simulink model "Environment_per_immagini_TESI"  (R2023a)
settings: Solver=FixedStepAuto  StartTime=0.0  StopTime=inf  RelTol=1e-3
values from neighbouring files (symbols this model uses):
  traiettoria = [x', y']    [generatoreTraiettoria.m]    (also in generatoreTraiettoria2.m; tra3.m)
undefined symbols (not defined in the file or in its folder): a, e1_0, p, Vdes
libraries: simulink x2, rllib x1
settings Model: Creator=Luzi  LastModifiedBy=Luzi

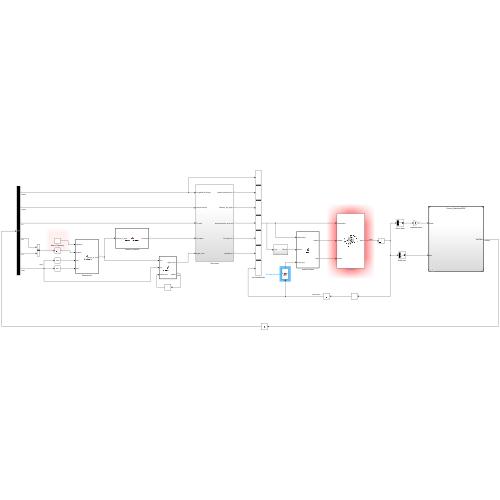
[thumbnail: Simulink's stored preview of the top-level diagram]
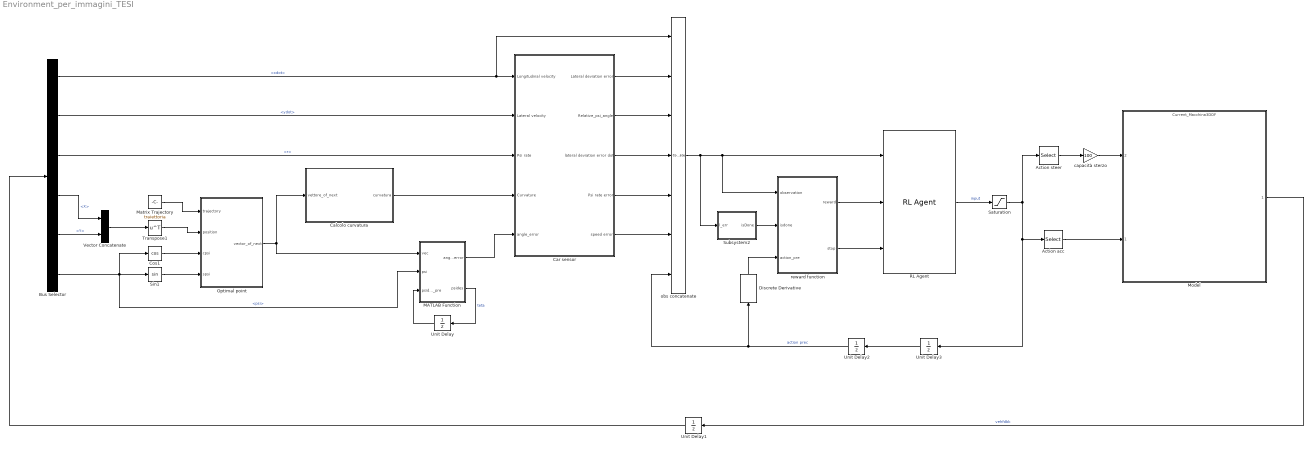
== system Environment_per_immagini_TESI ==
  Action acc : Selector  InputPortWidth=2  IndexOptions=Index vector (dialog)  Indices=2  OutputSizes=1
  Action steer : Selector  InputPortWidth=2  IndexOptions=Index vector (dialog)  Indices=1  OutputSizes=1
  Bus Selector : BusSelector  OutputSignals=BdyFrm.Cg.Vel.xdot,BdyFrm.Cg.Vel.ydot,BdyFrm.Cg.AngVel.r,InertFrm.Cg.Disp.X,InertFrm.Cg.Disp.Y,InertFrm.Cg.Ang.psi
  Calcolo curvatura : MATLAB Function  TreatAsAtomicUnit=on
  Car sensor : Subsystem
  Cos1 : Trigonometry  Operator=cos
  Discrete Derivative : simulink/Discrete/Discrete Derivative  gainval=0.1  ICPrevScaledInput=0.0  OutMin=[]  OutMax=[]  OutDataType=fixdt(1, 16)  OutScaling=2^-10  DoSatur=off
  MATLAB Function : MATLAB Function  TreatAsAtomicUnit=on
  Matrix Trajectory : Constant  Value=traiettoria  SampleTime=60
  Model : ModelReference  ModelNameDialog=Current_Macchina3DOF.slx  SimulationMode=Normal  ModelReferenceVersion=1.71
      settings: PortSchema="{\"entries\":[{\"content\":{\"sides\":[{\"content\":{\"connectorIds\":[\"In2\",\"In1\"]},\"type\":\"ConnectorPlacement.EquallySpacedRectSide\",\"uuid\":\"b5a44853-6584-4a50-847d-9a0b1c5ea9ac\"},{\"content\":{\"connectorIds\":[\"Out1\"],\"side\":\"RIGHT\"},\"type\":\"ConnectorPlacement.EquallySpacedRectSide\",\"uuid\":\"bfcb6c88-1d93-4f70-bf16-2c719fa247ba\"},{\"content\":{\"side\":\"TOP\"},\"type\":\"ConnectorPlacement.EquallySpacedRectSide\",\"uuid\":\"3385b00b-6ed4-40a5-8204-01acdd431cf5\"}]},\"type\":\"ConnectorPlacement.EquallySpacedConnector\",\"uuid\":\"3bb36942-6fbc-4d27-a33b-ca1de48b267b\"}],\"packageUris\":[\"http://schema.mathworks.com/mf0/Connector/R2020b\"],\"version\":\"1.0\"}"
  Optimal point : MATLAB Function  TreatAsAtomicUnit=on
  RL Agent : rllib/RL Agent  Agent=agent  ExternalActionAsInput=off  ProvideLastAction=off  ProvideCumRwd=off  TreatAsDirectFeedthrough=on  UseStrictObservationDataTypes=off
  Saturation : Saturate  UpperLimit=1  LowerLimit=-1
  Sin1 : Trigonometry
  Subsystem2 : Subsystem
  Transpose1 : Math  Operator=transpose
  Unit Delay{,1..3} (4 alike) : UnitDelay  SampleTime=-1  HasFrameUpgradeWarning=on
  Vector Concatenate : Concatenate
  capacità sterzo : Gain  Gain=100
  obs concatenate : Concatenate  NumInputs=7
  reward function : MATLAB Function  TreatAsAtomicUnit=on
  wires:
  Saturation/1 -> Action steer/1, Unit Delay3/1, Action acc/1
  Bus Selector/1 -> obs concatenate/1, Car sensor/1(Longitudinal velocity)  "<xdot>"
  Action steer/1 -> capacità sterzo/1
  obs concatenate/1 -> Subsystem2/1(l_err), reward function/1(observation), RL Agent/1
  RL Agent/1 -> Saturation/1  "input"
  Action acc/1 -> Model/1
  Bus Selector/2 -> Car sensor/2(Lateral velocity)  "<ydot>"
  Bus Selector/3 -> Car sensor/3(Psi rate)  "<r>"
  Calcolo curvatura/1(curvatura) -> Car sensor/4(Curvature)
  MATLAB Function/1(angle_error) -> Car sensor/5(angle_error)
  Unit Delay2/1 -> Discrete Derivative/1, obs concatenate/7  "action prec"
  Car sensor/5(speed error) -> obs concatenate/6
  Car sensor/4(Psi rate error) -> obs concatenate/5
  Car sensor/3(lateral deviation error dot) -> obs concatenate/4
  Car sensor/2(Relative_psi_angle) -> obs concatenate/3
  Car sensor/1(Lateral deviation error) -> obs concatenate/2
  MATLAB Function/2(psides) -> Unit Delay/1  "teta"
  Unit Delay/1 -> MATLAB Function/3(psides_pre)
  Optimal point/1(vector_of_next) -> Calcolo curvatura/1(vettore_of_next), MATLAB Function/1(vec)
  capacità sterzo/1 -> Model/2
  Model/1 -> Unit Delay1/1  "vehfdbk"
  Cos1/1 -> Optimal point/3(cpsi)
  Vector Concatenate/1 -> Transpose1/1
  Matrix Trajectory/1 -> Optimal point/1(trajectory)
  Bus Selector/6 -> MATLAB Function/2(psi), Sin1/1, Cos1/1  "<psi>"
  Sin1/1 -> Optimal point/4(spsi)
  Transpose1/1 -> Optimal point/2(position)
  Bus Selector/4 -> Vector Concatenate/1  "<X>"
  Bus Selector/5 -> Vector Concatenate/2  "<Y>"
  Subsystem2/1(isDone) -> reward function/2(isdone)
  reward function/2(stop) -> RL Agent/3
  reward function/1(reward) -> RL Agent/2
  Discrete Derivative/1 -> reward function/3(action_pre)
  Unit Delay1/1 -> Bus Selector/1
  Unit Delay3/1 -> Unit Delay2/1

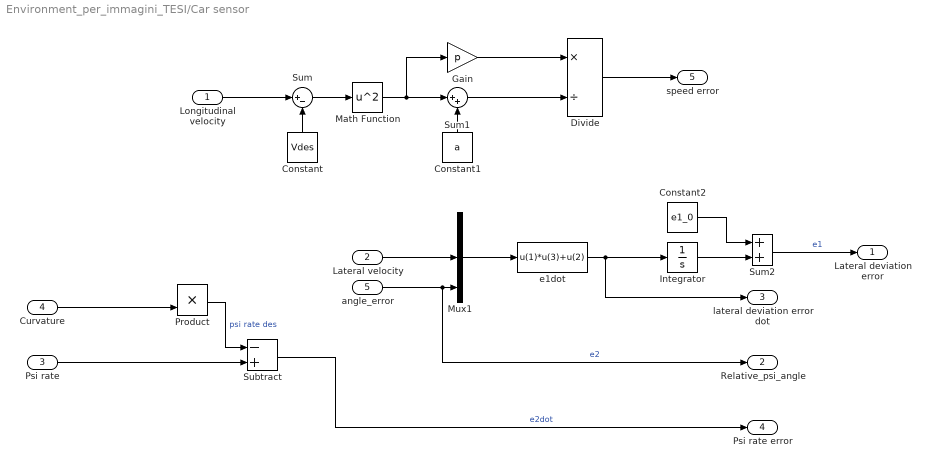
== system Environment_per_immagini_TESI/Car sensor ==
  Longitudinal velocity : Inport
  Lateral velocity : Inport  Port=2
  Psi rate : Inport  Port=3
  Curvature : Inport  Port=4
  angle_error : Inport  Port=5
  Constant : Constant  Value=Vdes
  Constant1 : Constant  Value=a
  Constant2 : Constant  Value=e1_0
  Divide : Product  Inputs=*/
  Gain : Gain  Gain=p
  Integrator : Integrator
  Math Function : Math  Operator=square
  Mux1 : Mux  Inputs=[1 1 1]
  Product : Product
  Subtract : Sum  Inputs=-+
  Sum : Sum  Inputs=|+-
  Sum1 : Sum  Inputs=|++
  Sum2 : Sum
  e1dot : Fcn  Expr=u(1)*u(3)+u(2)
  Lateral deviation error : Outport  VectorParamsAs1DForOutWhenUnconnected=off
  Relative_psi_angle : Outport  Port=2
  lateral deviation error dot : Outport  Port=3  VectorParamsAs1DForOutWhenUnconnected=off
  Psi rate error : Outport  Port=4  VectorParamsAs1DForOutWhenUnconnected=off
  speed error : Outport  Port=5
  wires:
  Curvature/1 -> Product/2
  Mux1/1 -> e1dot/1
  e1dot/1 -> lateral deviation error dot/1, Integrator/1
  Lateral velocity/1 -> Mux1/2
  Product/1 -> Subtract/1  "psi rate des"
  Psi rate/1 -> Subtract/2
  Subtract/1 -> Psi rate error/1  "e2dot"
  angle_error/1 -> Relative_psi_angle/1, Mux1/3  "e2"
  Constant/1 -> Sum/2
  Sum/1 -> Math Function/1
  Longitudinal velocity/1 -> Sum/1
  Math Function/1 -> Gain/1, Sum1/1
  Constant1/1 -> Sum1/2
  Sum1/1 -> Divide/2
  Gain/1 -> Divide/1
  Divide/1 -> speed error/1
  Integrator/1 -> Sum2/2
  Sum2/1 -> Lateral deviation error/1  "e1"
  Constant2/1 -> Sum2/1

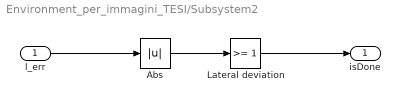
== system Environment_per_immagini_TESI/Subsystem2 ==
  l_err : Inport
  Abs : Abs  SaturateOnIntegerOverflow=off
  Lateral deviation : simulink/Logic and Bit Operations/Compare To Constant  relop=>=  const=1  OutDataTypeStr=boolean
  isDone : Outport  VectorParamsAs1DForOutWhenUnconnected=off
  wires:
  Abs/1 -> Lateral deviation/1
  l_err/1 -> Abs/1
  Lateral deviation/1 -> isDone/1

== matlab function Environment_per_immagini_TESI/MATLAB Function ==
  data: vec input; psi input; angle_error output; psides output; psides_pre input
function [angle_error,psides] = calc_angle_error(vec,psi, psides_pre)
    x1=vec(1,1);
    y1=vec(1,2);
    x3=vec(3,1);
    y3=vec(3,2);
    psides=atan2((y3-y1),(x3-x1));


     if(abs(tetapre-psides)>pi/4 && abs(tetapre-psides)<1.1*pi)%ATTENZIONE: PROVVISORIO PER RISOLVERE IL PROBLEMA DELL'INCROCIO DI TRAIETTORIE
         psides=tetapre;
     end



    angle_error=psi-psides;
    if angle_error>pi
        angle_error=angle_error-2*pi;
    elseif angle_error<-pi
        angle_error=angle_error+2*pi;
    end
end

== matlab function Environment_per_immagini_TESI/reward function ==
  data: observation input; isdone input; action_pre input; reward output; stop output
function [reward, stop] = reward(observation, isdone, action_pre)
    % Input:
    %   observation: vector containing relevant state information
    %   isdone: flag indicating whether the episode is finished
    %   action: vector representing the action taken
    %   action_d: vector representing the action derivatives
    % Output:
    %   speed_error: computed speed error based on the current velocity
    %   reward: calculated reward value considering various factors
    %   stop: flag indicating whether the episode should stop

    % Apply bonus based on lateral deviation
    
    if (e1^2 < 0.04)
        bonus_pos = 2;
    end

    if (e1^2 < 0.01)
        bonus_pos = bonus_pos + 0.5;
    end

    % Calculate the reward value
    reward = -(2 * e1^2 + 0.5*e2^2) - 50 * isdone + bonus_pos - speed_error - 0.25 * a_dot^2 - 1 * s_dot^2;

    stop = isdone;
end

%funzione countorf(x,y,z) per mappatura ricompenra e colorbar da inserire
%(nel editor matlab) per il controllo funzionalità

== matlab function Environment_per_immagini_TESI/Optimal point ==
  data: trajectory input; position input; cpsi input; spsi input; vector_of_next output
function vector_of_next  = optimalpoint(trajectory, position, cpsi, spsi)
    % Input:
    %   trajectory: Nx2 matrix representing the trajectory points
    %   position: 1x2 row vector representing the current position (xy)
    %   cpsi, spsi: components of the velocity direction
    % Output:
    %   point: 1x2 row vector representing the optimal point on the trajectory
    %   vector_of_next: 3x2 matrix containing the optimal point and the next two points

    % Initialize the matrix for the next points
    vector_of_next = zeros(3, 2);

    % Calculate distances between the current position and points on the trajectory
    N = size(trajectory, 1);
    distanceVector = zeros(N, 2);
    distanceValue = zeros(N, 1);

    for i = 1:N
        distanceVector(i, :) = trajectory(i, :) - position;
        distanceValue(i) = sqrt(distanceVector(i, 1)^2 + distanceVector(i, 2)^2);
    end

    % Find indices of the three nearest points
    [~, indx] = mink(distanceValue, 3);

    % Normalize distances and velocity direction
    distance1norm = distanceVector(indx(1), :) / norm(distanceVector(indx(1), :));
    distance2norm = distanceVector(indx(2), :) / norm(distanceVector(indx(2), :));
    distance3norm = distanceVector(indx(3), :) / norm(distanceVector(indx(3), :));
    direction = [cpsi, spsi];
    velocitynorm = direction;

    % Calculate dot product between normalized distances and velocity direction
    dotmatrix = [dot(distance1norm, velocitynorm), dot(distance2norm, velocitynorm), dot(distance3norm, velocitynorm)];

    % Find the index of the maximum dot product
    [~, I] = max(dotmatrix);

    % Get the optimal point

    if(indx(I)==1)
        vector_of_next(1,:)=point;
    else   
        vector_of_next(1,:)=trajectory(indx(I)-1,:);
    end

    vector_of_next(2,:)=point;

    if(indx(I)==length(trajectory))
        vector_of_next(3,:)=point;
    else
        vector_of_next(3,:)=trajectory(indx(I)+1,:);
    end
end

== matlab function Environment_per_immagini_TESI/Calcolo curvatura ==
  data: vettore_of_next input; curvatura output
function curvatura = calcola_curvatura(vettore_of_next)
    % Input:
    %   vettore_of_next: 3x2 matrix containing three points on the curve
    % Output:
    %   curvatura: vector containing the calculated curvature values

    % Extract x and y coordinates from the curve points
    x = vettore_of_next(:, 1);
    y = vettore_of_next(:, 2);

    % Calculate the first derivatives of x and y
    dx = diff(x);
    dy = diff(y);

    % Calculate the second derivatives of x and y
    d2x = diff(dx);
    d2y = diff(dy);

    % Calculate curvature using the formula: curvature = (dx * d2y - dy * d2x) / (dx^2 + dy^2)^(3/2)
    numeratore = dx(2:end) .* d2y - dy(2:end) .* d2x;
    denominatore = (dx(2:end).^2 + dy(2:end).^2).^(3/2);
    curvatura = numeratore ./ denominatore;

    % Handle any NaN values by setting them to zero
    for i = 1:length(curvatura)
        if (isnan(curvatura(i)))
            curvatura(i) = 0;
        end
    end
end
